simulink model "exp2_szm"  (R2019a)
settings: Solver=VariableStepAuto  StartTime=0.0  StopTime=10.0  RelTol=1e-3
libraries: truetime x2
settings Model: Creator=17827  LastModifiedBy=17827

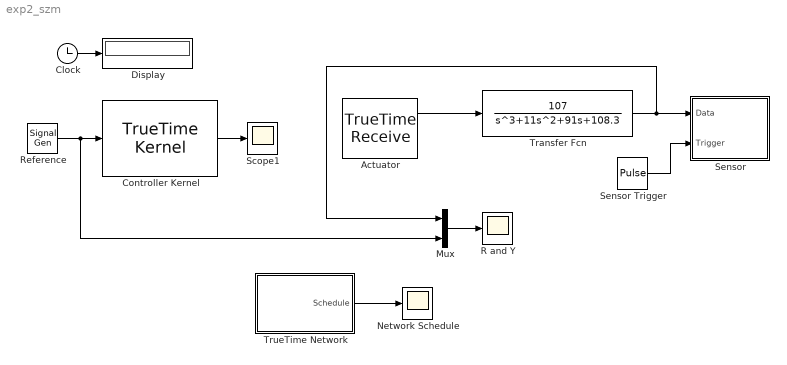
== system exp2_szm ==
  Actuator : truetime/TrueTime Receive  nwnbr=1  receiver=2  outdim=1  triggeroutput=on  senderoutput=off  lengthoutput=off  priorityoutput=off  timestampoutput=off  signalpoweroutput=off  msgIDoutput=off
  Clock : Clock
  Controller Kernel : truetime/TrueTime Kernel  sfun=node_init  args=[]  ninputsoutputs=[1 0]  ntriggers=0  trigtype=falling  nwnodenbr=1  clockoffsetdrift=[0 0]  schedoutput=on  battery=off  poweroutput=off  label=1: 1
  Display : Display
  Mux : Mux  Inputs=2
  Network Schedule : Scope
  R and Y : Scope
  Reference : SignalGenerator  WaveForm=square
  Scope1 : Scope
  Sensor : Subsystem  AncestorBlock=truetime/TrueTime Send  mask{trigger=falling, nwnbr=1, sender=2, indim=1, recsource=internal, receiver=1, lengthsource=internal, length=1000, priosource=internal, prio=1, msgIDsource=internal, msgID=0, dynamicSegment=dynamic}
      mask prompts: trigger "Trigger type:"; nwnbr "Network number:"; sender "Sender id:"; indim "Data input port dimension:"; recsource "Receiver source:"; receiver "Receiver id:"; lengthsource "Length source:"; length "Data length (bits):"; priosource "Priority source:"; prio "Priority (for CAN):"; msgIDsource "Message ID source:"; msgID "Message ID:"; dynamicSegment "Segment (for FlexRay):"
      mask init:
      | ttsend_callback(gcb,trigger,nwnbr,sender,recsource,lengthsource,priosource,msgIDsource)
      mask TypeOptions trigger: rising | falling | either
      mask TypeOptions recsource: internal | external
      mask Callback recsource: ttsend_callback
      mask TypeOptions lengthsource: internal | external
      mask Callback lengthsource: ttsend_callback
      mask TypeOptions priosource: internal | external
      mask Callback priosource: ttsend_callback
      mask TypeOptions msgIDsource: internal | external
      mask Callback msgIDsource: ttsend_callback
      mask TypeOptions dynamicSegment: static | dynamic
      mask Display: disp([num2str(nwnbr) ': ' num2str(sender)])
  Sensor Trigger : DiscretePulseGenerator  PulseType=Time based  Period=1  PulseWidth=5
  Transfer Fcn : TransferFcn  Numerator=[107]  Denominator=[1 11 91 108.3]
  TrueTime Network : Subsystem  AncestorBlock=truetime/TrueTime Network  mask(Real-Time Network){nwtype=CSMA/AMP (CAN), nwnbr=1, nnodes=2, rate=80, minsize=512, lossprob=0, seed=0, bandwidths=[0.5 0.5], slotsize=512, schedule=[1 1 2], memsize=80000, buftype=Common buffer, overflow=Retransmit, dynSchedule=0, miniSlotSize=0, NIT=0, QSortMode=FIFO, sync=0, irtSchedule=0, nrtLength=0, nodeGraph=0, scheduleoutput=on}
      mask prompts: nwtype "Network type:"; nwnbr "Network number:"; nnodes "Number of nodes:"; rate "Data rate (bits/s):"; minsize "Minimum frame size (bits):"; lossprob "Loss probability (0-1):"; seed "Initial seed:"; bandwidths "Bandwidth allocations:"; slotsize "Slotsize (bits):"; schedule "Static schedule:"; memsize "Total switch memory (bits):"; buftype "Switch buffer type:"; overflow "Switch overflow behavior:"; dynSchedule "Dynamic Schedule:"; miniSlotSize "Mini slot size (bits):"; NIT "Network idle time (bits):"; QSortMode "Input Queue Sorted by:"; sync "Synchronization length (bits):"; irtSchedule "IRT Schedule [msgID from to start arrival]:"; nrtLength "RT Class 1/NRT length (bits):"; nodeGraph "Node connection graph (nbrOfnodes x nbrOfNodes):"; scheduleoutput "Show Schedule output port:"
      mask init:
      | ttnetwork_callback(gcb,nwnbr,nnodes,scheduleoutput)
      mask TypeOptions nwtype: CSMA/CD (Ethernet) | CSMA/AMP (CAN) | Round Robin | FDMA | TDMA | Switched Ethernet | FlexRay | PROFINET | NCM
      mask Callback nwtype: ttnetwork_callback
      mask TypeOptions buftype: Common buffer | Symmetric output buffers
      mask TypeOptions overflow: Retransmit | Drop
      mask TypeOptions QSortMode: FIFO | Priority
      mask Display: disp(nwnbr)
  wires:
  Actuator/1 -> Transfer Fcn/1
  Transfer Fcn/1 -> Mux/1, Sensor/1(Data)
  Sensor Trigger/1 -> Sensor/2(Trigger)
  Clock/1 -> Display/1
  Controller Kernel/1 -> Scope1/1
  Reference/1 -> Mux/2, Controller Kernel/1
  TrueTime Network/1(Schedule) -> Network Schedule/1
  Mux/1 -> R and Y/1

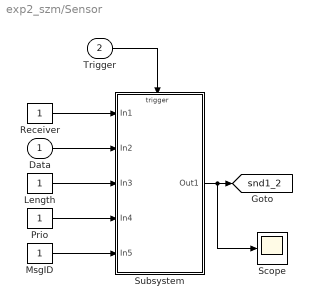
== system exp2_szm/Sensor ==
  Data : Inport
  Trigger : Inport  Port=2
  Length : Constant
  MsgID : Constant
  Prio : Constant
  Receiver : Constant
  Scope : Scope
  Subsystem : Subsystem  TreatAsAtomicUnit=on
  tag scope: snd1_2=global
  wires:
  Prio/1 -> Subsystem/4(In4)
  Length/1 -> Subsystem/3(In3)
  Receiver/1 -> Subsystem/1(In1)
  Data/1 -> Subsystem/2(In2)
  Subsystem/1(Out1) -> Scope/1, [snd1_2]
  Trigger/1 -> Subsystem/Trigger
  MsgID/1 -> Subsystem/5(In5)

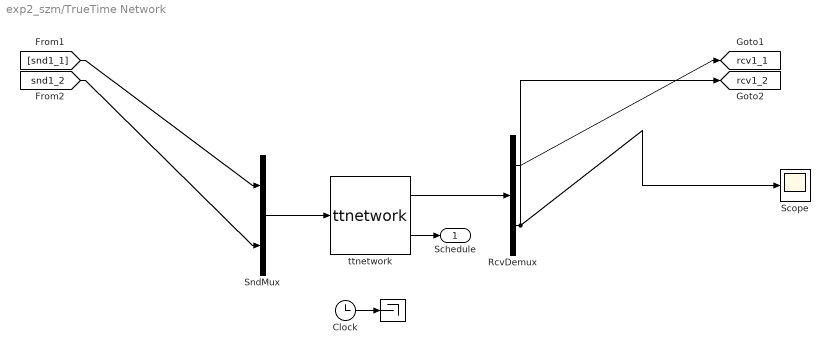
== system exp2_szm/TrueTime Network ==
  " " : Terminator
  Clock : Clock
  RcvDemux : Demux  Outputs=2
  Scope : Scope
  SndMux : Mux  Inputs=2
  ttnetwork : S-Function  FunctionName=ttnetwork  Parameters=nwtype,nwnbr,nnodes,rate,minsize,lossprob,bandwidths,slotsize,schedule,memsize,buftype,overflow,seed,dynSchedule,miniSlotSize,NIT,QSortMode,sync,irtSchedule,nrtLength,nodeGraph  SFunctionDeploymentMode=off  EnableBusSupport=off
  Schedule : Outport
  tag scope: rcv1_1=global, rcv1_2=global
  wires:
  Clock/1 -> " "/1
  SndMux/1 -> ttnetwork/1
  ttnetwork/1 -> RcvDemux/1
  ttnetwork/2 -> Schedule/1
  RcvDemux/2 -> Scope/1, [rcv1_2]
  [snd1_1] -> SndMux/1
  [snd1_2] -> SndMux/2
  RcvDemux/1 -> [rcv1_1]

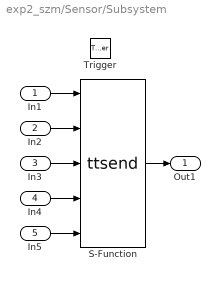
== system exp2_szm/Sensor/Subsystem ==
  In1 : Inport
  In2 : Inport  Port=2
  In3 : Inport  Port=3
  In4 : Inport  Port=4
  In5 : Inport  Port=5
  Trigger : TriggerPort  TriggerType=falling  VariantControl=(inherit)
  S-Function : S-Function  FunctionName=ttsend  Parameters=nwnbr,sender,indim,dynamicSegment  SFunctionDeploymentMode=off  EnableBusSupport=off
  Out1 : Outport
  wires:
  In1/1 -> S-Function/1
  In2/1 -> S-Function/2
  S-Function/1 -> Out1/1
  In3/1 -> S-Function/3
  In4/1 -> S-Function/4
  In5/1 -> S-Function/5
